simulink model "Nov_27"  (R2022a)
settings: Solver=FixedStepAuto  StartTime=0.0  StopTime=60  FixedStep=1e-3  RelTol=1e-3  EnableMultiTasking=on
undefined symbols (not defined in the file): D0, D1, D10, D11, D12, D13, D2, D3, D4, D5, D6, D7, D8, D9, PTA0, PTA1, PTA2, PTB23, PTB9, PTC16, PTC17, PTC2, PTC3, PTC4, PTD0, PTD1, PTD2, PTD3
libraries: frdmk64flib x16, etargetslib x1
(part 2 of 3)

== stateflow chart Nov_27/Requirements Table ==
  (default) -> (junction 1073743821)
  (junction 1073743821) -> (junction 1073743822) : {
      | % SF_REQ_REV_07
      | }
  (junction 1073743822) -> (junction 1073743824) : {
      | % HEADER_ASSIGNMENTS
      |
      | }
  (junction 1073743824) -> (junction 1073743826) : {
      | % START_A_4
      | }
  (junction 1073743826) -> (junction 1073743828) : {
      | }
  (junction 1073743828) -> (junction 1073743830)
  (junction 1073743830) -> (junction 1073743832) : {
      | }
  (junction 1073743832) -> (junction 1073743834) : {
      | % END_A_4
      | }
  (junction 1073743834) -> (junction 1073743836) : {
      | % START_R_1
      | }
  (junction 1073743836) -> (junction 1073743838) : {
      | }
  (junction 1073743838) -> (junction 1073743840)
  (junction 1073743840) -> (junction 1073743842) [order 1] : [((~((prev(ATR_GND_CTRL)) == (-100.0)))) && ((~((prev(ATR_PACE_CTRL)) == (-100.0)))) && ((~((prev(VENT_PACE_CTRL)) == (-100.0)))) && ((~((prev(VENT_GND_CTRL)) == (-100.0)))) && ((~((prev(PACE_CHARGE_CTRL)) == (-100.0)))) && ((~((VENT_CMP_DETECT) == (true)))) && ((~((ATR_CMP_DETECT) == (true)))) && ((~((VRP) == (-100)))) && (((ARP) == (150)) || ((ARP) == (160)) || ((ARP) == (170)) || ((ARP) == (180)) || ((ARP) == (190)) || ((ARP) == (200)) || ((ARP) == (210)) || ((ARP) == (220)) || ((ARP) == (230)) || ((ARP) == (240)) || ((ARP) == (250)) || ((ARP) == (260)) || ((ARP) == (270)) || ((ARP) == (280)) || ((ARP) == (290)) || ((ARP) == (300)) || ((ARP) == (310)) || ((ARP) == (320)) || ((ARP) == (330)) || ((ARP) == (340)) || ((ARP) == (350)) || ((ARP) == (360)) || ((ARP) == (370)) || ((ARP) == (380)) || ((ARP) == (390)) || ((ARP) == (400)) || ((ARP) == (410)) || ((ARP) == (420)) || ((ARP) == (430)) || ((ARP) == (440)) || ((ARP) == (450)) || ((ARP) == (460)) || ((ARP) == (470)) || ((ARP) == (480)) || ((ARP) == (490)) || ((ARP) == (500))) && (((URL_RATE_LIMIT) == (50)) || ((URL_RATE_LIMIT) == (55)) || ((URL_RATE_LIMIT) == (60)) || ((URL_RATE_LIMIT) == (65)) || ((URL_RATE_LIMIT) == (70)) || ((URL_RATE_LIMIT) == (75)) || ((URL_RATE_LIMIT) == (80)) || ((URL_RATE_LIMIT) == (85)) || ((URL_RATE_LIMIT) == (90)) || ((URL_RATE_LIMIT) == (95)) || ((URL_RATE_LIMIT) == (100)) || ((URL_RATE_LIMIT) == (105)) || ((URL_RATE_LIMIT) == (110)) || ((URL_RATE_LIMIT) == (115)) || ((URL_RATE_LIMIT) == (120)) || ((URL_RATE_LIMIT) == (125)) || ((URL_RATE_LIMIT) == (130)) || ((URL_RATE_LIMIT) == (135)) || ((URL_RATE_LIMIT) == (140)) || ((URL_RATE_LIMIT) == (145)) || ((URL_RATE_LIMIT) == (150)) || ((URL_RATE_LIMIT) == (155)) || ((URL_RATE_LIMIT) == (160)) || ((URL_RATE_LIMIT) == (165)) || ((URL_RATE_LIMIT) == (170)) || ((URL_RATE_LIMIT) == (175))) && (((ATR_PULSE_WIDTH) == (0.05)) || ((ATR_PULSE_WIDTH) == (0.1)) || ((ATR_PULSE_WIDTH) == (0.2)) || ((ATR_PULSE_WIDTH) == (0.3)) || ((ATR_PULSE_WIDTH) == (0.4)) || ((ATR_PULSE_WIDTH) == (0.5)) || ((ATR_PULSE_WIDTH) == (0.6)) || ((ATR_PULSE_WIDTH) == (0.7)) || ((ATR_PULSE_WIDTH) == (0.8)) || ((ATR_PULSE_WIDTH) == (0.9)) || ((ATR_PULSE_WIDTH) == (1)) || ((ATR_PULSE_WIDTH) == (1.1)) || ((ATR_PULSE_WIDTH) == (1.2)) || ((ATR_PULSE_WIDTH) == (1.3)) || ((ATR_PULSE_WIDTH) == (1.4)) || ((ATR_PULSE_WIDTH) == (1.5)) || ((ATR_PULSE_WIDTH) == (1.6)) || ((ATR_PULSE_WIDTH) == (1.7)) || ((ATR_PULSE_WIDTH) == (1.8)) || ((ATR_PULSE_WIDTH) == (1.9))) && ((~((VENT_PULSE_WIDTH) == (-100)))) && (((LRL_RATE_LIMIT) == (30)) || ((LRL_RATE_LIMIT) == (35)) || ((LRL_RATE_LIMIT) == (40)) || ((LRL_RATE_LIMIT) == (45)) || ((LRL_RATE_LIMIT) == (50)) || ((LRL_RATE_LIMIT) == (51)) || ((LRL_RATE_LIMIT) == (52)) || ((LRL_RATE_LIMIT) == (53)) || ((LRL_RATE_LIMIT) == (54)) || ((LRL_RATE_LIMIT) == (55)) || ((LRL_RATE_LIMIT) == (56)) || ((LRL_RATE_LIMIT) == (57)) || ((LRL_RATE_LIMIT) == (58)) || ((LRL_RATE_LIMIT) == (59)) || ((LRL_RATE_LIMIT) == (60)) || ((LRL_RATE_LIMIT) == (61)) || ((LRL_RATE_LIMIT) == (62)) || ((LRL_RATE_LIMIT) == (63)) || ((LRL_RATE_LIMIT) == (64)) || ((LRL_RATE_LIMIT) == (65)) || ((LRL_RATE_LIMIT) == (66)) || ((LRL_RATE_LIMIT) == (67)) || ((LRL_RATE_LIMIT) == (68)) || ((LRL_RATE_LIMIT) == (69)) || ((LRL_RATE_LIMIT) == (70)) || ((LRL_RATE_LIMIT) == (71)) || ((LRL_RATE_LIMIT) == (72)) || ((LRL_RATE_LIMIT) == (73)) || ((LRL_RATE_LIMIT) == (74)) || ((LRL_RATE_LIMIT) == (75)) || ((LRL_RATE_LIMIT) == (76)) || ((LRL_RATE_LIMIT) == (77)) || ((LRL_RATE_LIMIT) == (78)) || ((LRL_RATE_LIMIT) == (79)) || ((LRL_RATE_LIMIT) == (80)) || ((LRL_RATE_LIMIT) == (81)) || ((LRL_RATE_LIMIT) == (82)) || ((LRL_RATE_LIMIT) == (83)) || ((LRL_RATE_LIMIT) == (84)) || ((LRL_RATE_LIMIT) == (85)) || ((LRL_RATE_LIMIT) == (86)) || ((LRL_RATE_LIMIT) == (87)) || ((LRL_RATE_LIMIT) == (88)) || ((LRL_RATE_LIMIT) == (89)) || ((LRL_RATE_LIMIT) == (90)) || ((LRL_RATE_LIMIT) == (95)) || ((LRL_RATE_LIMIT) == (100)) || ((LRL_RATE_LIMIT) == (105)) || ((LRL_RATE_LIMIT) == (110)) || ((LRL_RATE_LIMIT) == (115)) || ((LRL_RATE_LIMIT) == (120)) || ((LRL_RATE_LIMIT) == (125)) || ((LRL_RATE_LIMIT) == (130)) || ((LRL_RATE_LIMIT) == (135)) || ((LRL_RATE_LIMIT) == (140)) || ((LRL_RATE_LIMIT) == (145)) || ((LRL_RATE_LIMIT) == (150)) || ((LRL_RATE_LIMIT) == (155)) || ((LRL_RATE_LIMIT) == (160)) || ((LRL_RATE_LIMIT) == (165)) || ((LRL_RATE_LIMIT) == (170)) || ((LRL_RATE_LIMIT) == (175)))]
  (junction 1073743840) -> (junction 1073743908) [order 2]
  (junction 1073743842) -> (junction 1073743844) : {
      | reqtable_postcondition(((~((ATR_GND_CTRL) == (-100.0)))) && ((~((ATR_PACE_CTRL) == (-100.0)))) && ((~((VENT_PACE_CTRL) == (-100.0)))) && ((~((VENT_GND_CTRL) == (-100.0)))) && ((~((PACE_CHARGE_CTRL) == (-100.0)))), 'R:1');
      |
      |
      | }
  (junction 1073743844) -> (junction 1073743846) : {
      | }
  (junction 1073743846) -> (junction 1073743848) : {
      | sf_internal_execute_R_31 = true;
      | }
  (junction 1073743848) -> (junction 1073743850) : {
      | % START_R_19
      | }
  (junction 1073743850) -> (junction 1073743852) : {
      | }
  (junction 1073743852) -> (junction 1073743854)
  (junction 1073743854) -> (junction 1073743856) [order 1] : [(((prev(ATR_GND_CTRL)) == (true))) && (((prev(ATR_PACE_CTRL)) == (false))) && (((prev(VENT_PACE_CTRL)) == (false))) && (((prev(VENT_GND_CTRL)) == (false))) && (((prev(PACE_CHARGE_CTRL)) == (true))) && ((~((VENT_CMP_DETECT) == (true)))) && ((~((ATR_CMP_DETECT) == (true)))) && ((~((VRP) == (-100)))) && (((ARP) == (150)) || ((ARP) == (160)) || ((ARP) == (170)) || ((ARP) == (180)) || ((ARP) == (190)) || ((ARP) == (200)) || ((ARP) == (210)) || ((ARP) == (220)) || ((ARP) == (230)) || ((ARP) == (240)) || ((ARP) == (250)) || ((ARP) == (260)) || ((ARP) == (270)) || ((ARP) == (280)) || ((ARP) == (290)) || ((ARP) == (300)) || ((ARP) == (310)) || ((ARP) == (320)) || ((ARP) == (330)) || ((ARP) == (340)) || ((ARP) == (350)) || ((ARP) == (360)) || ((ARP) == (370)) || ((ARP) == (380)) || ((ARP) == (390)) || ((ARP) == (400)) || ((ARP) == (410)) || ((ARP) == (420)) || ((ARP) == (430)) || ((ARP) == (440)) || ((ARP) == (450)) || ((ARP) == (460)) || ((ARP) == (470)) || ((ARP) == (480)) || ((ARP) == (490)) || ((ARP) == (500))) && (((URL_RATE_LIMIT) == (50)) || ((URL_RATE_LIMIT) == (55)) || ((URL_RATE_LIMIT) == (60)) || ((URL_RATE_LIMIT) == (65)) || ((URL_RATE_LIMIT) == (70)) || ((URL_RATE_LIMIT) == (75)) || ((URL_RATE_LIMIT) == (80)) || ((URL_RATE_LIMIT) == (85)) || ((URL_RATE_LIMIT) == (90)) || ((URL_RATE_LIMIT) == (95)) || ((URL_RATE_LIMIT) == (100)) || ((URL_RATE_LIMIT) == (105)) || ((URL_RATE_LIMIT) == (110)) || ((URL_RATE_LIMIT) == (115)) || ((URL_RATE_LIMIT) == (120)) || ((URL_RATE_LIMIT) == (125)) || ((URL_RATE_LIMIT) == (130)) || ((URL_RATE_LIMIT) == (135)) || ((URL_RATE_LIMIT) == (140)) || ((URL_RATE_LIMIT) == (145)) || ((URL_RATE_LIMIT) == (150)) || ((URL_RATE_LIMIT) == (155)) || ((URL_RATE_LIMIT) == (160)) || ((URL_RATE_LIMIT) == (165)) || ((URL_RATE_LIMIT) == (170)) || ((URL_RATE_LIMIT) == (175))) && (((ATR_PULSE_WIDTH) == (0.05)) || ((ATR_PULSE_WIDTH) == (0.1)) || ((ATR_PULSE_WIDTH) == (0.2)) || ((ATR_PULSE_WIDTH) == (0.3)) || ((ATR_PULSE_WIDTH) == (0.4)) || ((ATR_PULSE_WIDTH) == (0.5)) || ((ATR_PULSE_WIDTH) == (0.6)) || ((ATR_PULSE_WIDTH) == (0.7)) || ((ATR_PULSE_WIDTH) == (0.8)) || ((ATR_PULSE_WIDTH) == (0.9)) || ((ATR_PULSE_WIDTH) == (1)) || ((ATR_PULSE_WIDTH) == (1.1)) || ((ATR_PULSE_WIDTH) == (1.2)) || ((ATR_PULSE_WIDTH) == (1.3)) || ((ATR_PULSE_WIDTH) == (1.4)) || ((ATR_PULSE_WIDTH) == (1.5)) || ((ATR_PULSE_WIDTH) == (1.6)) || ((ATR_PULSE_WIDTH) == (1.7)) || ((ATR_PULSE_WIDTH) == (1.8)) || ((ATR_PULSE_WIDTH) == (1.9))) && ((~((VENT_PULSE_WIDTH) == (-100)))) && (((LRL_RATE_LIMIT) == (30)) || ((LRL_RATE_LIMIT) == (35)) || ((LRL_RATE_LIMIT) == (40)) || ((LRL_RATE_LIMIT) == (45)) || ((LRL_RATE_LIMIT) == (50)) || ((LRL_RATE_LIMIT) == (51)) || ((LRL_RATE_LIMIT) == (52)) || ((LRL_RATE_LIMIT) == (53)) || ((LRL_RATE_LIMIT) == (54)) || ((LRL_RATE_LIMIT) == (55)) || ((LRL_RATE_LIMIT) == (56)) || ((LRL_RATE_LIMIT) == (57)) || ((LRL_RATE_LIMIT) == (58)) || ((LRL_RATE_LIMIT) == (59)) || ((LRL_RATE_LIMIT) == (60)) || ((LRL_RATE_LIMIT) == (61)) || ((LRL_RATE_LIMIT) == (62)) || ((LRL_RATE_LIMIT) == (63)) || ((LRL_RATE_LIMIT) == (64)) || ((LRL_RATE_LIMIT) == (65)) || ((LRL_RATE_LIMIT) == (66)) || ((LRL_RATE_LIMIT) == (67)) || ((LRL_RATE_LIMIT) == (68)) || ((LRL_RATE_LIMIT) == (69)) || ((LRL_RATE_LIMIT) == (70)) || ((LRL_RATE_LIMIT) == (71)) || ((LRL_RATE_LIMIT) == (72)) || ((LRL_RATE_LIMIT) == (73)) || ((LRL_RATE_LIMIT) == (74)) || ((LRL_RATE_LIMIT) == (75)) || ((LRL_RATE_LIMIT) == (76)) || ((LRL_RATE_LIMIT) == (77)) || ((LRL_RATE_LIMIT) == (78)) || ((LRL_RATE_LIMIT) == (79)) || ((LRL_RATE_LIMIT) == (80)) || ((LRL_RATE_LIMIT) == (81)) || ((LRL_RATE_LIMIT) == (82)) || ((LRL_RATE_LIMIT) == (83)) || ((LRL_RATE_LIMIT) == (84)) || ((LRL_RATE_LIMIT) == (85)) || ((LRL_RATE_LIMIT) == (86)) || ((LRL_RATE_LIMIT) == (87)) || ((LRL_RATE_LIMIT) == (88)) || ((LRL_RATE_LIMIT) == (89)) || ((LRL_RATE_LIMIT) == (90)) || ((LRL_RATE_LIMIT) == (95)) || ((LRL_RATE_LIMIT) == (100)) || ((LRL_RATE_LIMIT) == (105)) || ((LRL_RATE_LIMIT) == (110)) || ((LRL_RATE_LIMIT) == (115)) || ((LRL_RATE_LIMIT) == (120)) || ((LRL_RATE_LIMIT) == (125)) || ((LRL_RATE_LIMIT) == (130)) || ((LRL_RATE_LIMIT) == (135)) || ((LRL_RATE_LIMIT) == (140)) || ((LRL_RATE_LIMIT) == (145)) || ((LRL_RATE_LIMIT) == (150)) || ((LRL_RATE_LIMIT) == (155)) || ((LRL_RATE_LIMIT) == (160)) || ((LRL_RATE_LIMIT) == (165)) || ((LRL_RATE_LIMIT) == (170)) || ((LRL_RATE_LIMIT) == (175)))]
  (junction 1073743854) -> (junction 1073743864) [order 2]
  (junction 1073743856) -> (junction 1073743858) : {
      | reqtable_postcondition((((ATR_GND_CTRL) == (false))) && (((ATR_PACE_CTRL) == (true))) && (((VENT_PACE_CTRL) == (false))) && (((VENT_GND_CTRL) == (false))) && (((PACE_CHARGE_CTRL) == (false))), 'R:1.1');
      |
      |
      | }
  (junction 1073743858) -> (junction 1073743860) : {
      | }
  (junction 1073743860) -> (junction 1073743862) : {
      | sf_internal_execute_R_31 = false;
      | }
  (junction 1073743862) -> (junction 1073743864)
  (junction 1073743864) -> (junction 1073743866)
  (junction 1073743866) -> (junction 1073743868) : {
      | % END_R_19
      | }
  (junction 1073743868) -> (junction 1073743870) : {
      | % START_R_22
      | }
  (junction 1073743870) -> (junction 1073743872) : {
      | }
  (junction 1073743872) -> (junction 1073743874)
  (junction 1073743874) -> (junction 1073743876) [order 1] : [(((prev(ATR_GND_CTRL)) == (true || false))) && (((prev(ATR_PACE_CTRL)) == (true || false))) && (((prev(VENT_PACE_CTRL)) == (false))) && (((prev(VENT_GND_CTRL)) == (false))) && (((prev(PACE_CHARGE_CTRL)) == (true || false))) && ((~((VENT_CMP_DETECT) == (true)))) && (((ATR_CMP_DETECT) == (true))) && ((~((VRP) == (-100)))) && (((ARP) == (150)) || ((ARP) == (160)) || ((ARP) == (170)) || ((ARP) == (180)) || ((ARP) == (190)) || ((ARP) == (200)) || ((ARP) == (210)) || ((ARP) == (220)) || ((ARP) == (230)) || ((ARP) == (240)) || ((ARP) == (250)) || ((ARP) == (260)) || ((ARP) == (270)) || ((ARP) == (280)) || ((ARP) == (290)) || ((ARP) == (300)) || ((ARP) == (310)) || ((ARP) == (320)) || ((ARP) == (330)) || ((ARP) == (340)) || ((ARP) == (350)) || ((ARP) == (360)) || ((ARP) == (370)) || ((ARP) == (380)) || ((ARP) == (390)) || ((ARP) == (400)) || ((ARP) == (410)) || ((ARP) == (420)) || ((ARP) == (430)) || ((ARP) == (440)) || ((ARP) == (450)) || ((ARP) == (460)) || ((ARP) == (470)) || ((ARP) == (480)) || ((ARP) == (490)) || ((ARP) == (500))) && (((URL_RATE_LIMIT) == (50)) || ((URL_RATE_LIMIT) == (55)) || ((URL_RATE_LIMIT) == (60)) || ((URL_RATE_LIMIT) == (65)) || ((URL_RATE_LIMIT) == (70)) || ((URL_RATE_LIMIT) == (75)) || ((URL_RATE_LIMIT) == (80)) || ((URL_RATE_LIMIT) == (85)) || ((URL_RATE_LIMIT) == (90)) || ((URL_RATE_LIMIT) == (95)) || ((URL_RATE_LIMIT) == (100)) || ((URL_RATE_LIMIT) == (105)) || ((URL_RATE_LIMIT) == (110)) || ((URL_RATE_LIMIT) == (115)) || ((URL_RATE_LIMIT) == (120)) || ((URL_RATE_LIMIT) == (125)) || ((URL_RATE_LIMIT) == (130)) || ((URL_RATE_LIMIT) == (135)) || ((URL_RATE_LIMIT) == (140)) || ((URL_RATE_LIMIT) == (145)) || ((URL_RATE_LIMIT) == (150)) || ((URL_RATE_LIMIT) == (155)) || ((URL_RATE_LIMIT) == (160)) || ((URL_RATE_LIMIT) == (165)) || ((URL_RATE_LIMIT) == (170)) || ((URL_RATE_LIMIT) == (175))) && (((ATR_PULSE_WIDTH) == (0.05)) || ((ATR_PULSE_WIDTH) == (0.1)) || ((ATR_PULSE_WIDTH) == (0.2)) || ((ATR_PULSE_WIDTH) == (0.3)) || ((ATR_PULSE_WIDTH) == (0.4)) || ((ATR_PULSE_WIDTH) == (0.5)) || ((ATR_PULSE_WIDTH) == (0.6)) || ((ATR_PULSE_WIDTH) == (0.7)) || ((ATR_PULSE_WIDTH) == (0.8)) || ((ATR_PULSE_WIDTH) == (0.9)) || ((ATR_PULSE_WIDTH) == (1)) || ((ATR_PULSE_WIDTH) == (1.1)) || ((ATR_PULSE_WIDTH) == (1.2)) || ((ATR_PULSE_WIDTH) == (1.3)) || ((ATR_PULSE_WIDTH) == (1.4)) || ((ATR_PULSE_WIDTH) == (1.5)) || ((ATR_PULSE_WIDTH) == (1.6)) || ((ATR_PULSE_WIDTH) == (1.7)) || ((ATR_PULSE_WIDTH) == (1.8)) || ((ATR_PULSE_WIDTH) == (1.9))) && ((~((VENT_PULSE_WIDTH) == (-100)))) && (((LRL_RATE_LIMIT) == (30)) || ((LRL_RATE_LIMIT) == (35)) || ((LRL_RATE_LIMIT) == (40)) || ((LRL_RATE_LIMIT) == (45)) || ((LRL_RATE_LIMIT) == (50)) || ((LRL_RATE_LIMIT) == (51)) || ((LRL_RATE_LIMIT) == (52)) || ((LRL_RATE_LIMIT) == (53)) || ((LRL_RATE_LIMIT) == (54)) || ((LRL_RATE_LIMIT) == (55)) || ((LRL_RATE_LIMIT) == (56)) || ((LRL_RATE_LIMIT) == (57)) || ((LRL_RATE_LIMIT) == (58)) || ((LRL_RATE_LIMIT) == (59)) || ((LRL_RATE_LIMIT) == (60)) || ((LRL_RATE_LIMIT) == (61)) || ((LRL_RATE_LIMIT) == (62)) || ((LRL_RATE_LIMIT) == (63)) || ((LRL_RATE_LIMIT) == (64)) || ((LRL_RATE_LIMIT) == (65)) || ((LRL_RATE_LIMIT) == (66)) || ((LRL_RATE_LIMIT) == (67)) || ((LRL_RATE_LIMIT) == (68)) || ((LRL_RATE_LIMIT) == (69)) || ((LRL_RATE_LIMIT) == (70)) || ((LRL_RATE_LIMIT) == (71)) || ((LRL_RATE_LIMIT) == (72)) || ((LRL_RATE_LIMIT) == (73)) || ((LRL_RATE_LIMIT) == (74)) || ((LRL_RATE_LIMIT) == (75)) || ((LRL_RATE_LIMIT) == (76)) || ((LRL_RATE_LIMIT) == (77)) || ((LRL_RATE_LIMIT) == (78)) || ((LRL_RATE_LIMIT) == (79)) || ((LRL_RATE_LIMIT) == (80)) || ((LRL_RATE_LIMIT) == (81)) || ((LRL_RATE_LIMIT) == (82)) || ((LRL_RATE_LIMIT) == (83)) || ((LRL_RATE_LIMIT) == (84)) || ((LRL_RATE_LIMIT) == (85)) || ((LRL_RATE_LIMIT) == (86)) || ((LRL_RATE_LIMIT) == (87)) || ((LRL_RATE_LIMIT) == (88)) || ((LRL_RATE_LIMIT) == (89)) || ((LRL_RATE_LIMIT) == (90)) || ((LRL_RATE_LIMIT) == (95)) || ((LRL_RATE_LIMIT) == (100)) || ((LRL_RATE_LIMIT) == (105)) || ((LRL_RATE_LIMIT) == (110)) || ((LRL_RATE_LIMIT) == (115)) || ((LRL_RATE_LIMIT) == (120)) || ((LRL_RATE_LIMIT) == (125)) || ((LRL_RATE_LIMIT) == (130)) || ((LRL_RATE_LIMIT) == (135)) || ((LRL_RATE_LIMIT) == (140)) || ((LRL_RATE_LIMIT) == (145)) || ((LRL_RATE_LIMIT) == (150)) || ((LRL_RATE_LIMIT) == (155)) || ((LRL_RATE_LIMIT) == (160)) || ((LRL_RATE_LIMIT) == (165)) || ((LRL_RATE_LIMIT) == (170)) || ((LRL_RATE_LIMIT) == (175)))]
  (junction 1073743874) -> (junction 1073743884) [order 2]
  (junction 1073743876) -> (junction 1073743878) : {
      | reqtable_postcondition((((ATR_GND_CTRL) == (true))) && (((ATR_PACE_CTRL) == (false))) && (((VENT_PACE_CTRL) == (false))) && (((VENT_GND_CTRL) == (false))) && (((PACE_CHARGE_CTRL) == (true))), 'R:1.2');
      |
      |
      | }
  (junction 1073743878) -> (junction 1073743880) : {
      | }
  (junction 1073743880) -> (junction 1073743882) : {
      | sf_internal_execute_R_31 = false;
      | }
  (junction 1073743882) -> (junction 1073743884)
  (junction 1073743884) -> (junction 1073743886)
  (junction 1073743886) -> (junction 1073743888) : {
      | % END_R_22
      | }
  (junction 1073743888) -> (junction 1073743890) : {
      | % START_R_31
      | }
  (junction 1073743890) -> (junction 1073743892) : {
      | }
  (junction 1073743892) -> (junction 1073743894)
  (junction 1073743894) -> (junction 1073743896) [order 1] : [sf_internal_execute_R_31]
  (junction 1073743894) -> (junction 1073743902) [order 2]
  (junction 1073743896) -> (junction 1073743898) : {
      | reqtable_postcondition((((ATR_GND_CTRL) == (true))) && (((ATR_PACE_CTRL) == (false))) && (((VENT_PACE_CTRL) == (false))) && (((VENT_GND_CTRL) == (false))) && (((PACE_CHARGE_CTRL) == (true))), 'R:1.3');
      |
      |
      | }
  (junction 1073743898) -> (junction 1073743900) : {
      | }
  (junction 1073743900) -> (junction 1073743902)
  (junction 1073743902) -> (junction 1073743904)
  (junction 1073743904) -> (junction 1073743906) : {
      | % END_R_31
      | }
  (junction 1073743906) -> (junction 1073743908)
  (junction 1073743908) -> (junction 1073743910)
  (junction 1073743910) -> (junction 1073743912) : {
      | % END_R_1
      | }
  (junction 1073743912) -> (junction 1073743914) : {
      | % START_R_34
      | }
  (junction 1073743914) -> (junction 1073743916) : {
      | }
  (junction 1073743916) -> (junction 1073743918)
  (junction 1073743918) -> (junction 1073743920) [order 1] : [((~((prev(ATR_GND_CTRL)) == (-100.0)))) && ((~((prev(ATR_PACE_CTRL)) == (-100.0)))) && ((~((prev(VENT_PACE_CTRL)) == (-100.0)))) && ((~((prev(VENT_GND_CTRL)) == (-100.0)))) && ((~((prev(PACE_CHARGE_CTRL)) == (-100.0)))) && ((~((VENT_CMP_DETECT) == (true)))) && ((~((ATR_CMP_DETECT) == (true)))) && (((VRP) == (150)) || ((VRP) == (160)) || ((VRP) == (170)) || ((VRP) == (180)) || ((VRP) == (190)) || ((VRP) == (200)) || ((VRP) == (210)) || ((VRP) == (220)) || ((VRP) == (230)) || ((VRP) == (240)) || ((VRP) == (250)) || ((VRP) == (260)) || ((VRP) == (270)) || ((VRP) == (280)) || ((VRP) == (290)) || ((VRP) == (300)) || ((VRP) == (310)) || ((VRP) == (320)) || ((VRP) == (330)) || ((VRP) == (340)) || ((VRP) == (350)) || ((VRP) == (360)) || ((VRP) == (370)) || ((VRP) == (380)) || ((VRP) == (390)) || ((VRP) == (400)) || ((VRP) == (410)) || ((VRP) == (420)) || ((VRP) == (430)) || ((VRP) == (440)) || ((VRP) == (450)) || ((VRP) == (460)) || ((VRP) == (470)) || ((VRP) == (480)) || ((VRP) == (490)) || ((VRP) == (500))) && ((~((ARP) == (-100)))) && (((URL_RATE_LIMIT) == (50)) || ((URL_RATE_LIMIT) == (55)) || ((URL_RATE_LIMIT) == (60)) || ((URL_RATE_LIMIT) == (65)) || ((URL_RATE_LIMIT) == (70)) || ((URL_RATE_LIMIT) == (75)) || ((URL_RATE_LIMIT) == (80)) || ((URL_RATE_LIMIT) == (85)) || ((URL_RATE_LIMIT) == (90)) || ((URL_RATE_LIMIT) == (95)) || ((URL_RATE_LIMIT) == (100)) || ((URL_RATE_LIMIT) == (105)) || ((URL_RATE_LIMIT) == (110)) || ((URL_RATE_LIMIT) == (115)) || ((URL_RATE_LIMIT) == (120)) || ((URL_RATE_LIMIT) == (125)) || ((URL_RATE_LIMIT) == (130)) || ((URL_RATE_LIMIT) == (135)) || ((URL_RATE_LIMIT) == (140)) || ((URL_RATE_LIMIT) == (145)) || ((URL_RATE_LIMIT) == (150)) || ((URL_RATE_LIMIT) == (155)) || ((URL_RATE_LIMIT) == (160)) || ((URL_RATE_LIMIT) == (165)) || ((URL_RATE_LIMIT) == (170)) || ((URL_RATE_LIMIT) == (175))) && ((~((ATR_PULSE_WIDTH) == (-100)))) && (((VENT_PULSE_WIDTH) == (0.05)) || ((VENT_PULSE_WIDTH) == (0.1)) || ((VENT_PULSE_WIDTH) == (0.2)) || ((VENT_PULSE_WIDTH) == (0.3)) || ((VENT_PULSE_WIDTH) == (0.4)) || ((VENT_PULSE_WIDTH) == (0.5)) || ((VENT_PULSE_WIDTH) == (0.6)) || ((VENT_PULSE_WIDTH) == (0.7)) || ((VENT_PULSE_WIDTH) == (0.8)) || ((VENT_PULSE_WIDTH) == (0.9)) || ((VENT_PULSE_WIDTH) == (1)) || ((VENT_PULSE_WIDTH) == (1.1)) || ((VENT_PULSE_WIDTH) == (1.2)) || ((VENT_PULSE_WIDTH) == (1.3)) || ((VENT_PULSE_WIDTH) == (1.4)) || ((VENT_PULSE_WIDTH) == (1.5)) || ((VENT_PULSE_WIDTH) == (1.6)) || ((VENT_PULSE_WIDTH) == (1.7)) || ((VENT_PULSE_WIDTH) == (1.8)) || ((VENT_PULSE_WIDTH) == (1.9))) && (((LRL_RATE_LIMIT) == (30)) || ((LRL_RATE_LIMIT) == (35)) || ((LRL_RATE_LIMIT) == (40)) || ((LRL_RATE_LIMIT) == (45)) || ((LRL_RATE_LIMIT) == (50)) || ((LRL_RATE_LIMIT) == (51)) || ((LRL_RATE_LIMIT) == (52)) || ((LRL_RATE_LIMIT) == (53)) || ((LRL_RATE_LIMIT) == (54)) || ((LRL_RATE_LIMIT) == (55)) || ((LRL_RATE_LIMIT) == (56)) || ((LRL_RATE_LIMIT) == (57)) || ((LRL_RATE_LIMIT) == (58)) || ((LRL_RATE_LIMIT) == (59)) || ((LRL_RATE_LIMIT) == (60)) || ((LRL_RATE_LIMIT) == (61)) || ((LRL_RATE_LIMIT) == (62)) || ((LRL_RATE_LIMIT) == (63)) || ((LRL_RATE_LIMIT) == (64)) || ((LRL_RATE_LIMIT) == (65)) || ((LRL_RATE_LIMIT) == (66)) || ((LRL_RATE_LIMIT) == (67)) || ((LRL_RATE_LIMIT) == (68)) || ((LRL_RATE_LIMIT) == (69)) || ((LRL_RATE_LIMIT) == (70)) || ((LRL_RATE_LIMIT) == (71)) || ((LRL_RATE_LIMIT) == (72)) || ((LRL_RATE_LIMIT) == (73)) || ((LRL_RATE_LIMIT) == (74)) || ((LRL_RATE_LIMIT) == (75)) || ((LRL_RATE_LIMIT) == (76)) || ((LRL_RATE_LIMIT) == (77)) || ((LRL_RATE_LIMIT) == (78)) || ((LRL_RATE_LIMIT) == (79)) || ((LRL_RATE_LIMIT) == (80)) || ((LRL_RATE_LIMIT) == (81)) || ((LRL_RATE_LIMIT) == (82)) || ((LRL_RATE_LIMIT) == (83)) || ((LRL_RATE_LIMIT) == (84)) || ((LRL_RATE_LIMIT) == (85)) || ((LRL_RATE_LIMIT) == (86)) || ((LRL_RATE_LIMIT) == (87)) || ((LRL_RATE_LIMIT) == (88)) || ((LRL_RATE_LIMIT) == (89)) || ((LRL_RATE_LIMIT) == (90)) || ((LRL_RATE_LIMIT) == (95)) || ((LRL_RATE_LIMIT) == (100)) || ((LRL_RATE_LIMIT) == (105)) || ((LRL_RATE_LIMIT) == (110)) || ((LRL_RATE_LIMIT) == (115)) || ((LRL_RATE_LIMIT) == (120)) || ((LRL_RATE_LIMIT) == (125)) || ((LRL_RATE_LIMIT) == (130)) || ((LRL_RATE_LIMIT) == (135)) || ((LRL_RATE_LIMIT) == (140)) || ((LRL_RATE_LIMIT) == (145)) || ((LRL_RATE_LIMIT) == (150)) || ((LRL_RATE_LIMIT) == (155)) || ((LRL_RATE_LIMIT) == (160)) || ((LRL_RATE_LIMIT) == (165)) || ((LRL_RATE_LIMIT) == (170)) || ((LRL_RATE_LIMIT) == (175)))]
  (junction 1073743918) -> (junction 1073743986) [order 2]
  (junction 1073743920) -> (junction 1073743922) : {
      | reqtable_postcondition(((~((ATR_GND_CTRL) == (-100.0)))) && ((~((ATR_PACE_CTRL) == (-100.0)))) && ((~((VENT_PACE_CTRL) == (-100.0)))) && ((~((VENT_GND_CTRL) == (-100.0)))) && ((~((PACE_CHARGE_CTRL) == (-100.0)))), 'R:2');
      |
      |
      | }
  (junction 1073743922) -> (junction 1073743924) : {
      | }
  (junction 1073743924) -> (junction 1073743926) : {
      | sf_internal_execute_R_46 = true;
      | }
  (junction 1073743926) -> (junction 1073743928) : {
      | % START_R_37
      | }
  (junction 1073743928) -> (junction 1073743930) : {
      | }
  (junction 1073743930) -> (junction 1073743932)
  (junction 1073743932) -> (junction 1073743934) [order 1] : [(((prev(ATR_GND_CTRL)) == (false))) && (((prev(ATR_PACE_CTRL)) == (false))) && (((prev(VENT_PACE_CTRL)) == (false))) && (((prev(VENT_GND_CTRL)) == (true))) && (((prev(PACE_CHARGE_CTRL)) == (true))) && ((~((VENT_CMP_DETECT) == (true)))) && ((~((ATR_CMP_DETECT) == (true)))) && (((VRP) == (150)) || ((VRP) == (160)) || ((VRP) == (170)) || ((VRP) == (180)) || ((VRP) == (190)) || ((VRP) == (200)) || ((VRP) == (210)) || ((VRP) == (220)) || ((VRP) == (230)) || ((VRP) == (240)) || ((VRP) == (250)) || ((VRP) == (260)) || ((VRP) == (270)) || ((VRP) == (280)) || ((VRP) == (290)) || ((VRP) == (300)) || ((VRP) == (310)) || ((VRP) == (320)) || ((VRP) == (330)) || ((VRP) == (340)) || ((VRP) == (350)) || ((VRP) == (360)) || ((VRP) == (370)) || ((VRP) == (380)) || ((VRP) == (390)) || ((VRP) == (400)) || ((VRP) == (410)) || ((VRP) == (420)) || ((VRP) == (430)) || ((VRP) == (440)) || ((VRP) == (450)) || ((VRP) == (460)) || ((VRP) == (470)) || ((VRP) == (480)) || ((VRP) == (490)) || ((VRP) == (500))) && ((~((ARP) == (-100)))) && (((URL_RATE_LIMIT) == (50)) || ((URL_RATE_LIMIT) == (55)) || ((URL_RATE_LIMIT) == (60)) || ((URL_RATE_LIMIT) == (65)) || ((URL_RATE_LIMIT) == (70)) || ((URL_RATE_LIMIT) == (75)) || ((URL_RATE_LIMIT) == (80)) || ((URL_RATE_LIMIT) == (85)) || ((URL_RATE_LIMIT) == (90)) || ((URL_RATE_LIMIT) == (95)) || ((URL_RATE_LIMIT) == (100)) || ((URL_RATE_LIMIT) == (105)) || ((URL_RATE_LIMIT) == (110)) || ((URL_RATE_LIMIT) == (115)) || ((URL_RATE_LIMIT) == (120)) || ((URL_RATE_LIMIT) == (125)) || ((URL_RATE_LIMIT) == (130)) || ((URL_RATE_LIMIT) == (135)) || ((URL_RATE_LIMIT) == (140)) || ((URL_RATE_LIMIT) == (145)) || ((URL_RATE_LIMIT) == (150)) || ((URL_RATE_LIMIT) == (155)) || ((URL_RATE_LIMIT) == (160)) || ((URL_RATE_LIMIT) == (165)) || ((URL_RATE_LIMIT) == (170)) || ((URL_RATE_LIMIT) == (175))) && ((~((ATR_PULSE_WIDTH) == (-100)))) && (((VENT_PULSE_WIDTH) == (0.05)) || ((VENT_PULSE_WIDTH) == (0.1)) || ((VENT_PULSE_WIDTH) == (0.2)) || ((VENT_PULSE_WIDTH) == (0.3)) || ((VENT_PULSE_WIDTH) == (0.4)) || ((VENT_PULSE_WIDTH) == (0.5)) || ((VENT_PULSE_WIDTH) == (0.6)) || ((VENT_PULSE_WIDTH) == (0.7)) || ((VENT_PULSE_WIDTH) == (0.8)) || ((VENT_PULSE_WIDTH) == (0.9)) || ((VENT_PULSE_WIDTH) == (1)) || ((VENT_PULSE_WIDTH) == (1.1)) || ((VENT_PULSE_WIDTH) == (1.2)) || ((VENT_PULSE_WIDTH) == (1.3)) || ((VENT_PULSE_WIDTH) == (1.4)) || ((VENT_PULSE_WIDTH) == (1.5)) || ((VENT_PULSE_WIDTH) == (1.6)) || ((VENT_PULSE_WIDTH) == (1.7)) || ((VENT_PULSE_WIDTH) == (1.8)) || ((VENT_PULSE_WIDTH) == (1.9))) && (((LRL_RATE_LIMIT) == (30)) || ((LRL_RATE_LIMIT) == (35)) || ((LRL_RATE_LIMIT) == (40)) || ((LRL_RATE_LIMIT) == (45)) || ((LRL_RATE_LIMIT) == (50)) || ((LRL_RATE_LIMIT) == (51)) || ((LRL_RATE_LIMIT) == (52)) || ((LRL_RATE_LIMIT) == (53)) || ((LRL_RATE_LIMIT) == (54)) || ((LRL_RATE_LIMIT) == (55)) || ((LRL_RATE_LIMIT) == (56)) || ((LRL_RATE_LIMIT) == (57)) || ((LRL_RATE_LIMIT) == (58)) || ((LRL_RATE_LIMIT) == (59)) || ((LRL_RATE_LIMIT) == (60)) || ((LRL_RATE_LIMIT) == (61)) || ((LRL_RATE_LIMIT) == (62)) || ((LRL_RATE_LIMIT) == (63)) || ((LRL_RATE_LIMIT) == (64)) || ((LRL_RATE_LIMIT) == (65)) || ((LRL_RATE_LIMIT) == (66)) || ((LRL_RATE_LIMIT) == (67)) || ((LRL_RATE_LIMIT) == (68)) || ((LRL_RATE_LIMIT) == (69)) || ((LRL_RATE_LIMIT) == (70)) || ((LRL_RATE_LIMIT) == (71)) || ((LRL_RATE_LIMIT) == (72)) || ((LRL_RATE_LIMIT) == (73)) || ((LRL_RATE_LIMIT) == (74)) || ((LRL_RATE_LIMIT) == (75)) || ((LRL_RATE_LIMIT) == (76)) || ((LRL_RATE_LIMIT) == (77)) || ((LRL_RATE_LIMIT) == (78)) || ((LRL_RATE_LIMIT) == (79)) || ((LRL_RATE_LIMIT) == (80)) || ((LRL_RATE_LIMIT) == (81)) || ((LRL_RATE_LIMIT) == (82)) || ((LRL_RATE_LIMIT) == (83)) || ((LRL_RATE_LIMIT) == (84)) || ((LRL_RATE_LIMIT) == (85)) || ((LRL_RATE_LIMIT) == (86)) || ((LRL_RATE_LIMIT) == (87)) || ((LRL_RATE_LIMIT) == (88)) || ((LRL_RATE_LIMIT) == (89)) || ((LRL_RATE_LIMIT) == (90)) || ((LRL_RATE_LIMIT) == (95)) || ((LRL_RATE_LIMIT) == (100)) || ((LRL_RATE_LIMIT) == (105)) || ((LRL_RATE_LIMIT) == (110)) || ((LRL_RATE_LIMIT) == (115)) || ((LRL_RATE_LIMIT) == (120)) || ((LRL_RATE_LIMIT) == (125)) || ((LRL_RATE_LIMIT) == (130)) || ((LRL_RATE_LIMIT) == (135)) || ((LRL_RATE_LIMIT) == (140)) || ((LRL_RATE_LIMIT) == (145)) || ((LRL_RATE_LIMIT) == (150)) || ((LRL_RATE_LIMIT) == (155)) || ((LRL_RATE_LIMIT) == (160)) || ((LRL_RATE_LIMIT) == (165)) || ((LRL_RATE_LIMIT) == (170)) || ((LRL_RATE_LIMIT) == (175)))]
  (junction 1073743932) -> (junction 1073743942) [order 2]
  (junction 1073743934) -> (junction 1073743936) : {
      | reqtable_postcondition((((ATR_GND_CTRL) == (false))) && (((ATR_PACE_CTRL) == (false))) && (((VENT_PACE_CTRL) == (true))) && (((VENT_GND_CTRL) == (false))) && (((PACE_CHARGE_CTRL) == (false))), 'R:2.1');
      |
      |
      | }
  (junction 1073743936) -> (junction 1073743938) : {
      | }
  (junction 1073743938) -> (junction 1073743940) : {
      | sf_internal_execute_R_46 = false;
      | }
  (junction 1073743940) -> (junction 1073743942)
  (junction 1073743942) -> (junction 1073743944)
  (junction 1073743944) -> (junction 1073743946) : {
      | % END_R_37
      | }
  (junction 1073743946) -> (junction 1073743948) : {
      | % START_R_43
      | }
  (junction 1073743948) -> (junction 1073743950) : {
      | }
  (junction 1073743950) -> (junction 1073743952)
  (junction 1073743952) -> (junction 1073743954) [order 1] : [(((prev(ATR_GND_CTRL)) == (false))) && (((prev(ATR_PACE_CTRL)) == (false))) && (((prev(VENT_PACE_CTRL)) == (true || false))) && (((prev(VENT_GND_CTRL)) == (true || false))) && (((prev(PACE_CHARGE_CTRL)) == (true || false))) && (((VENT_CMP_DETECT) == (true))) && ((~((ATR_CMP_DETECT) == (true)))) && (((VRP) == (150)) || ((VRP) == (160)) || ((VRP) == (170)) || ((VRP) == (180)) || ((VRP) == (190)) || ((VRP) == (200)) || ((VRP) == (210)) || ((VRP) == (220)) || ((VRP) == (230)) || ((VRP) == (240)) || ((VRP) == (250)) || ((VRP) == (260)) || ((VRP) == (270)) || ((VRP) == (280)) || ((VRP) == (290)) || ((VRP) == (300)) || ((VRP) == (310)) || ((VRP) == (320)) || ((VRP) == (330)) || ((VRP) == (340)) || ((VRP) == (350)) || ((VRP) == (360)) || ((VRP) == (370)) || ((VRP) == (380)) || ((VRP) == (390)) || ((VRP) == (400)) || ((VRP) == (410)) || ((VRP) == (420)) || ((VRP) == (430)) || ((VRP) == (440)) || ((VRP) == (450)) || ((VRP) == (460)) || ((VRP) == (470)) || ((VRP) == (480)) || ((VRP) == (490)) || ((VRP) == (500))) && ((~((ARP) == (-100)))) && (((URL_RATE_LIMIT) == (50)) || ((URL_RATE_LIMIT) == (55)) || ((URL_RATE_LIMIT) == (60)) || ((URL_RATE_LIMIT) == (65)) || ((URL_RATE_LIMIT) == (70)) || ((URL_RATE_LIMIT) == (75)) || ((URL_RATE_LIMIT) == (80)) || ((URL_RATE_LIMIT) == (85)) || ((URL_RATE_LIMIT) == (90)) || ((URL_RATE_LIMIT) == (95)) || ((URL_RATE_LIMIT) == (100)) || ((URL_RATE_LIMIT) == (105)) || ((URL_RATE_LIMIT) == (110)) || ((URL_RATE_LIMIT) == (115)) || ((URL_RATE_LIMIT) == (120)) || ((URL_RATE_LIMIT) == (125)) || ((URL_RATE_LIMIT) == (130)) || ((URL_RATE_LIMIT) == (135)) || ((URL_RATE_LIMIT) == (140)) || ((URL_RATE_LIMIT) == (145)) || ((URL_RATE_LIMIT) == (150)) || ((URL_RATE_LIMIT) == (155)) || ((URL_RATE_LIMIT) == (160)) || ((URL_RATE_LIMIT) == (165)) || ((URL_RATE_LIMIT) == (170)) || ((URL_RATE_LIMIT) == (175))) && ((~((ATR_PULSE_WIDTH) == (-100)))) && (((VENT_PULSE_WIDTH) == (0.05)) || ((VENT_PULSE_WIDTH) == (0.1)) || ((VENT_PULSE_WIDTH) == (0.2)) || ((VENT_PULSE_WIDTH) == (0.3)) || ((VENT_PULSE_WIDTH) == (0.4)) || ((VENT_PULSE_WIDTH) == (0.5)) || ((VENT_PULSE_WIDTH) == (0.6)) || ((VENT_PULSE_WIDTH) == (0.7)) || ((VENT_PULSE_WIDTH) == (0.8)) || ((VENT_PULSE_WIDTH) == (0.9)) || ((VENT_PULSE_WIDTH) == (1)) || ((VENT_PULSE_WIDTH) == (1.1)) || ((VENT_PULSE_WIDTH) == (1.2)) || ((VENT_PULSE_WIDTH) == (1.3)) || ((VENT_PULSE_WIDTH) == (1.4)) || ((VENT_PULSE_WIDTH) == (1.5)) || ((VENT_PULSE_WIDTH) == (1.6)) || ((VENT_PULSE_WIDTH) == (1.7)) || ((VENT_PULSE_WIDTH) == (1.8)) || ((VENT_PULSE_WIDTH) == (1.9))) && (((LRL_RATE_LIMIT) == (30)) || ((LRL_RATE_LIMIT) == (35)) || ((LRL_RATE_LIMIT) == (40)) || ((LRL_RATE_LIMIT) == (45)) || ((LRL_RATE_LIMIT) == (50)) || ((LRL_RATE_LIMIT) == (51)) || ((LRL_RATE_LIMIT) == (52)) || ((LRL_RATE_LIMIT) == (53)) || ((LRL_RATE_LIMIT) == (54)) || ((LRL_RATE_LIMIT) == (55)) || ((LRL_RATE_LIMIT) == (56)) || ((LRL_RATE_LIMIT) == (57)) || ((LRL_RATE_LIMIT) == (58)) || ((LRL_RATE_LIMIT) == (59)) || ((LRL_RATE_LIMIT) == (60)) || ((LRL_RATE_LIMIT) == (61)) || ((LRL_RATE_LIMIT) == (62)) || ((LRL_RATE_LIMIT) == (63)) || ((LRL_RATE_LIMIT) == (64)) || ((LRL_RATE_LIMIT) == (65)) || ((LRL_RATE_LIMIT) == (66)) || ((LRL_RATE_LIMIT) == (67)) || ((LRL_RATE_LIMIT) == (68)) || ((LRL_RATE_LIMIT) == (69)) || ((LRL_RATE_LIMIT) == (70)) || ((LRL_RATE_LIMIT) == (71)) || ((LRL_RATE_LIMIT) == (72)) || ((LRL_RATE_LIMIT) == (73)) || ((LRL_RATE_LIMIT) == (74)) || ((LRL_RATE_LIMIT) == (75)) || ((LRL_RATE_LIMIT) == (76)) || ((LRL_RATE_LIMIT) == (77)) || ((LRL_RATE_LIMIT) == (78)) || ((LRL_RATE_LIMIT) == (79)) || ((LRL_RATE_LIMIT) == (80)) || ((LRL_RATE_LIMIT) == (81)) || ((LRL_RATE_LIMIT) == (82)) || ((LRL_RATE_LIMIT) == (83)) || ((LRL_RATE_LIMIT) == (84)) || ((LRL_RATE_LIMIT) == (85)) || ((LRL_RATE_LIMIT) == (86)) || ((LRL_RATE_LIMIT) == (87)) || ((LRL_RATE_LIMIT) == (88)) || ((LRL_RATE_LIMIT) == (89)) || ((LRL_RATE_LIMIT) == (90)) || ((LRL_RATE_LIMIT) == (95)) || ((LRL_RATE_LIMIT) == (100)) || ((LRL_RATE_LIMIT) == (105)) || ((LRL_RATE_LIMIT) == (110)) || ((LRL_RATE_LIMIT) == (115)) || ((LRL_RATE_LIMIT) == (120)) || ((LRL_RATE_LIMIT) == (125)) || ((LRL_RATE_LIMIT) == (130)) || ((LRL_RATE_LIMIT) == (135)) || ((LRL_RATE_LIMIT) == (140)) || ((LRL_RATE_LIMIT) == (145)) || ((LRL_RATE_LIMIT) == (150)) || ((LRL_RATE_LIMIT) == (155)) || ((LRL_RATE_LIMIT) == (160)) || ((LRL_RATE_LIMIT) == (165)) || ((LRL_RATE_LIMIT) == (170)) || ((LRL_RATE_LIMIT) == (175)))]
  (junction 1073743952) -> (junction 1073743962) [order 2]
  (junction 1073743954) -> (junction 1073743956) : {
      | reqtable_postcondition((((ATR_GND_CTRL) == (false))) && (((ATR_PACE_CTRL) == (false))) && (((VENT_PACE_CTRL) == (false))) && (((VENT_GND_CTRL) == (true))) && (((PACE_CHARGE_CTRL) == (true))), 'R:2.2');
      |
      |
      | }
  (junction 1073743956) -> (junction 1073743958) : {
      | }
  (junction 1073743958) -> (junction 1073743960) : {
      | sf_internal_execute_R_46 = false;
      | }
  (junction 1073743960) -> (junction 1073743962)
  (junction 1073743962) -> (junction 1073743964)
  (junction 1073743964) -> (junction 1073743966) : {
      | % END_R_43
      | }
  (junction 1073743966) -> (junction 1073743968) : {
      | % START_R_46
      | }
  (junction 1073743968) -> (junction 1073743970) : {
      | }
  (junction 1073743970) -> (junction 1073743972)
  (junction 1073743972) -> (junction 1073743974) [order 1] : [sf_internal_execute_R_46]
  (junction 1073743972) -> (junction 1073743980) [order 2]
  (junction 1073743974) -> (junction 1073743976) : {
      | reqtable_postcondition((((ATR_GND_CTRL) == (false))) && (((ATR_PACE_CTRL) == (false))) && (((VENT_PACE_CTRL) == (false))) && (((VENT_GND_CTRL) == (true))) && (((PACE_CHARGE_CTRL) == (true))), 'R:2.3');
      |
      |
      | }
  (junction 1073743976) -> (junction 1073743978) : {
      | }
  (junction 1073743978) -> (junction 1073743980)
  (junction 1073743980) -> (junction 1073743982)
  (junction 1073743982) -> (junction 1073743984) : {
      | % END_R_46
      | }
  (junction 1073743984) -> (junction 1073743986)
  (junction 1073743986) -> (junction 1073743988)
  (junction 1073743988) -> (junction 1073743990) : {
      | % END_R_34
      | }
  (junction 1073743990) -> (junction 1073743992) : {
      | % START_R_49
      | }
  (junction 1073743992) -> (junction 1073743994) : {
      | }
  (junction 1073743994) -> (junction 1073743996)
  (junction 1073743996) -> (junction 1073743998) [order 1] : [((~((prev(ATR_GND_CTRL)) == (-100.0)))) && ((~((prev(ATR_PACE_CTRL)) == (-100.0)))) && ((~((prev(VENT_PACE_CTRL)) == (-100.0)))) && ((~((prev(VENT_GND_CTRL)) == (-100.0)))) && ((~((prev(PACE_CHARGE_CTRL)) == (-100.0)))) && ((~((VENT_CMP_DETECT) == (true)))) && ((~((ATR_CMP_DETECT) == (true)))) && ((~((VRP) == (-100)))) && ((~((ARP) == (-100)))) && (((URL_RATE_LIMIT) == (50)) || ((URL_RATE_LIMIT) == (55)) || ((URL_RATE_LIMIT) == (60)) || ((URL_RATE_LIMIT) == (65)) || ((URL_RATE_LIMIT) == (70)) || ((URL_RATE_LIMIT) == (75)) || ((URL_RATE_LIMIT) == (80)) || ((URL_RATE_LIMIT) == (85)) || ((URL_RATE_LIMIT) == (90)) || ((URL_RATE_LIMIT) == (95)) || ((URL_RATE_LIMIT) == (100)) || ((URL_RATE_LIMIT) == (105)) || ((URL_RATE_LIMIT) == (110)) || ((URL_RATE_LIMIT) == (115)) || ((URL_RATE_LIMIT) == (120)) || ((URL_RATE_LIMIT) == (125)) || ((URL_RATE_LIMIT) == (130)) || ((URL_RATE_LIMIT) == (135)) || ((URL_RATE_LIMIT) == (140)) || ((URL_RATE_LIMIT) == (145)) || ((URL_RATE_LIMIT) == (150)) || ((URL_RATE_LIMIT) == (155)) || ((URL_RATE_LIMIT) == (160)) || ((URL_RATE_LIMIT) == (165)) || ((URL_RATE_LIMIT) == (170)) || ((URL_RATE_LIMIT) == (175))) && ((~((ATR_PULSE_WIDTH) == (-100)))) && (((VENT_PULSE_WIDTH) == (0.05)) || ((VENT_PULSE_WIDTH) == (0.1)) || ((VENT_PULSE_WIDTH) == (0.2)) || ((VENT_PULSE_WIDTH) == (0.3)) || ((VENT_PULSE_WIDTH) == (0.4)) || ((VENT_PULSE_WIDTH) == (0.5)) || ((VENT_PULSE_WIDTH) == (0.6)) || ((VENT_PULSE_WIDTH) == (0.7)) || ((VENT_PULSE_WIDTH) == (0.8)) || ((VENT_PULSE_WIDTH) == (0.9)) || ((VENT_PULSE_WIDTH) == (1)) || ((VENT_PULSE_WIDTH) == (1.1)) || ((VENT_PULSE_WIDTH) == (1.2)) || ((VENT_PULSE_WIDTH) == (1.3)) || ((VENT_PULSE_WIDTH) == (1.4)) || ((VENT_PULSE_WIDTH) == (1.5)) || ((VENT_PULSE_WIDTH) == (1.6)) || ((VENT_PULSE_WIDTH) == (1.7)) || ((VENT_PULSE_WIDTH) == (1.8)) || ((VENT_PULSE_WIDTH) == (1.9))) && (((LRL_RATE_LIMIT) == (30)) || ((LRL_RATE_LIMIT) == (35)) || ((LRL_RATE_LIMIT) == (40)) || ((LRL_RATE_LIMIT) == (45)) || ((LRL_RATE_LIMIT) == (50)) || ((LRL_RATE_LIMIT) == (51)) || ((LRL_RATE_LIMIT) == (52)) || ((LRL_RATE_LIMIT) == (53)) || ((LRL_RATE_LIMIT) == (54)) || ((LRL_RATE_LIMIT) == (55)) || ((LRL_RATE_LIMIT) == (56)) || ((LRL_RATE_LIMIT) == (57)) || ((LRL_RATE_LIMIT) == (58)) || ((LRL_RATE_LIMIT) == (59)) || ((LRL_RATE_LIMIT) == (60)) || ((LRL_RATE_LIMIT) == (61)) || ((LRL_RATE_LIMIT) == (62)) || ((LRL_RATE_LIMIT) == (63)) || ((LRL_RATE_LIMIT) == (64)) || ((LRL_RATE_LIMIT) == (65)) || ((LRL_RATE_LIMIT) == (66)) || ((LRL_RATE_LIMIT) == (67)) || ((LRL_RATE_LIMIT) == (68)) || ((LRL_RATE_LIMIT) == (69)) || ((LRL_RATE_LIMIT) == (70)) || ((LRL_RATE_LIMIT) == (71)) || ((LRL_RATE_LIMIT) == (72)) || ((LRL_RATE_LIMIT) == (73)) || ((LRL_RATE_LIMIT) == (74)) || ((LRL_RATE_LIMIT) == (75)) || ((LRL_RATE_LIMIT) == (76)) || ((LRL_RATE_LIMIT) == (77)) || ((LRL_RATE_LIMIT) == (78)) || ((LRL_RATE_LIMIT) == (79)) || ((LRL_RATE_LIMIT) == (80)) || ((LRL_RATE_LIMIT) == (81)) || ((LRL_RATE_LIMIT) == (82)) || ((LRL_RATE_LIMIT) == (83)) || ((LRL_RATE_LIMIT) == (84)) || ((LRL_RATE_LIMIT) == (85)) || ((LRL_RATE_LIMIT) == (86)) || ((LRL_RATE_LIMIT) == (87)) || ((LRL_RATE_LIMIT) == (88)) || ((LRL_RATE_LIMIT) == (89)) || ((LRL_RATE_LIMIT) == (90)) || ((LRL_RATE_LIMIT) == (95)) || ((LRL_RATE_LIMIT) == (100)) || ((LRL_RATE_LIMIT) == (105)) || ((LRL_RATE_LIMIT) == (110)) || ((LRL_RATE_LIMIT) == (115)) || ((LRL_RATE_LIMIT) == (120)) || ((LRL_RATE_LIMIT) == (125)) || ((LRL_RATE_LIMIT) == (130)) || ((LRL_RATE_LIMIT) == (135)) || ((LRL_RATE_LIMIT) == (140)) || ((LRL_RATE_LIMIT) == (145)) || ((LRL_RATE_LIMIT) == (150)) || ((LRL_RATE_LIMIT) == (155)) || ((LRL_RATE_LIMIT) == (160)) || ((LRL_RATE_LIMIT) == (165)) || ((LRL_RATE_LIMIT) == (170)) || ((LRL_RATE_LIMIT) == (175)))]
  (junction 1073743996) -> (junction 1073744044) [order 2]
  (junction 1073743998) -> (junction 1073744000) : {
      | reqtable_postcondition(((~((ATR_GND_CTRL) == (-100.0)))) && ((~((ATR_PACE_CTRL) == (-100.0)))) && ((~((VENT_PACE_CTRL) == (-100.0)))) && ((~((VENT_GND_CTRL) == (-100.0)))) && ((~((PACE_CHARGE_CTRL) == (-100.0)))), 'R:3');
      |
      |
      | }
  (junction 1073744000) -> (junction 1073744002) : {
      | }
  (junction 1073744002) -> (junction 1073744004) : {
      | sf_internal_execute_R_55 = true;
      | }
  (junction 1073744004) -> (junction 1073744006) : {
      | % START_R_52
      | }
  (junction 1073744006) -> (junction 1073744008) : {
      | }
  (junction 1073744008) -> (junction 1073744010)
  (junction 1073744010) -> (junction 1073744012) [order 1] : [(((prev(ATR_GND_CTRL)) == (false))) && (((prev(ATR_PACE_CTRL)) == (false))) && (((prev(VENT_PACE_CTRL)) == (false))) && (((prev(VENT_GND_CTRL)) == (true))) && (((prev(PACE_CHARGE_CTRL)) == (true))) && ((~((VENT_CMP_DETECT) == (true)))) && ((~((ATR_CMP_DETECT) == (true)))) && ((~((VRP) == (-100)))) && ((~((ARP) == (-100)))) && (((URL_RATE_LIMIT) == (50)) || ((URL_RATE_LIMIT) == (55)) || ((URL_RATE_LIMIT) == (60)) || ((URL_RATE_LIMIT) == (65)) || ((URL_RATE_LIMIT) == (70)) || ((URL_RATE_LIMIT) == (75)) || ((URL_RATE_LIMIT) == (80)) || ((URL_RATE_LIMIT) == (85)) || ((URL_RATE_LIMIT) == (90)) || ((URL_RATE_LIMIT) == (95)) || ((URL_RATE_LIMIT) == (100)) || ((URL_RATE_LIMIT) == (105)) || ((URL_RATE_LIMIT) == (110)) || ((URL_RATE_LIMIT) == (115)) || ((URL_RATE_LIMIT) == (120)) || ((URL_RATE_LIMIT) == (125)) || ((URL_RATE_LIMIT) == (130)) || ((URL_RATE_LIMIT) == (135)) || ((URL_RATE_LIMIT) == (140)) || ((URL_RATE_LIMIT) == (145)) || ((URL_RATE_LIMIT) == (150)) || ((URL_RATE_LIMIT) == (155)) || ((URL_RATE_LIMIT) == (160)) || ((URL_RATE_LIMIT) == (165)) || ((URL_RATE_LIMIT) == (170)) || ((URL_RATE_LIMIT) == (175))) && ((~((ATR_PULSE_WIDTH) == (-100)))) && (((VENT_PULSE_WIDTH) == (0.05)) || ((VENT_PULSE_WIDTH) == (0.1)) || ((VENT_PULSE_WIDTH) == (0.2)) || ((VENT_PULSE_WIDTH) == (0.3)) || ((VENT_PULSE_WIDTH) == (0.4)) || ((VENT_PULSE_WIDTH) == (0.5)) || ((VENT_PULSE_WIDTH) == (0.6)) || ((VENT_PULSE_WIDTH) == (0.7)) || ((VENT_PULSE_WIDTH) == (0.8)) || ((VENT_PULSE_WIDTH) == (0.9)) || ((VENT_PULSE_WIDTH) == (1)) || ((VENT_PULSE_WIDTH) == (1.1)) || ((VENT_PULSE_WIDTH) == (1.2)) || ((VENT_PULSE_WIDTH) == (1.3)) || ((VENT_PULSE_WIDTH) == (1.4)) || ((VENT_PULSE_WIDTH) == (1.5)) || ((VENT_PULSE_WIDTH) == (1.6)) || ((VENT_PULSE_WIDTH) == (1.7)) || ((VENT_PULSE_WIDTH) == (1.8)) || ((VENT_PULSE_WIDTH) == (1.9))) && (((LRL_RATE_LIMIT) == (30)) || ((LRL_RATE_LIMIT) == (35)) || ((LRL_RATE_LIMIT) == (40)) || ((LRL_RATE_LIMIT) == (45)) || ((LRL_RATE_LIMIT) == (50)) || ((LRL_RATE_LIMIT) == (51)) || ((LRL_RATE_LIMIT) == (52)) || ((LRL_RATE_LIMIT) == (53)) || ((LRL_RATE_LIMIT) == (54)) || ((LRL_RATE_LIMIT) == (55)) || ((LRL_RATE_LIMIT) == (56)) || ((LRL_RATE_LIMIT) == (57)) || ((LRL_RATE_LIMIT) == (58)) || ((LRL_RATE_LIMIT) == (59)) || ((LRL_RATE_LIMIT) == (60)) || ((LRL_RATE_LIMIT) == (61)) || ((LRL_RATE_LIMIT) == (62)) || ((LRL_RATE_LIMIT) == (63)) || ((LRL_RATE_LIMIT) == (64)) || ((LRL_RATE_LIMIT) == (65)) || ((LRL_RATE_LIMIT) == (66)) || ((LRL_RATE_LIMIT) == (67)) || ((LRL_RATE_LIMIT) == (68)) || ((LRL_RATE_LIMIT) == (69)) || ((LRL_RATE_LIMIT) == (70)) || ((LRL_RATE_LIMIT) == (71)) || ((LRL_RATE_LIMIT) == (72)) || ((LRL_RATE_LIMIT) == (73)) || ((LRL_RATE_LIMIT) == (74)) || ((LRL_RATE_LIMIT) == (75)) || ((LRL_RATE_LIMIT) == (76)) || ((LRL_RATE_LIMIT) == (77)) || ((LRL_RATE_LIMIT) == (78)) || ((LRL_RATE_LIMIT) == (79)) || ((LRL_RATE_LIMIT) == (80)) || ((LRL_RATE_LIMIT) == (81)) || ((LRL_RATE_LIMIT) == (82)) || ((LRL_RATE_LIMIT) == (83)) || ((LRL_RATE_LIMIT) == (84)) || ((LRL_RATE_LIMIT) == (85)) || ((LRL_RATE_LIMIT) == (86)) || ((LRL_RATE_LIMIT) == (87)) || ((LRL_RATE_LIMIT) == (88)) || ((LRL_RATE_LIMIT) == (89)) || ((LRL_RATE_LIMIT) == (90)) || ((LRL_RATE_LIMIT) == (95)) || ((LRL_RATE_LIMIT) == (100)) || ((LRL_RATE_LIMIT) == (105)) || ((LRL_RATE_LIMIT) == (110)) || ((LRL_RATE_LIMIT) == (115)) || ((LRL_RATE_LIMIT) == (120)) || ((LRL_RATE_LIMIT) == (125)) || ((LRL_RATE_LIMIT) == (130)) || ((LRL_RATE_LIMIT) == (135)) || ((LRL_RATE_LIMIT) == (140)) || ((LRL_RATE_LIMIT) == (145)) || ((LRL_RATE_LIMIT) == (150)) || ((LRL_RATE_LIMIT) == (155)) || ((LRL_RATE_LIMIT) == (160)) || ((LRL_RATE_LIMIT) == (165)) || ((LRL_RATE_LIMIT) == (170)) || ((LRL_RATE_LIMIT) == (175)))]
  (junction 1073744010) -> (junction 1073744020) [order 2]
  (junction 1073744012) -> (junction 1073744014) : {
      | reqtable_postcondition((((ATR_GND_CTRL) == (false))) && (((ATR_PACE_CTRL) == (false))) && (((VENT_PACE_CTRL) == (true))) && (((VENT_GND_CTRL) == (false))) && (((PACE_CHARGE_CTRL) == (false))), 'R:3.1');
      |
      |
      | }
  (junction 1073744014) -> (junction 1073744016) : {
      | }
  (junction 1073744016) -> (junction 1073744018) : {
      | sf_internal_execute_R_55 = false;
      | }
  (junction 1073744018) -> (junction 1073744020)
  (junction 1073744020) -> (junction 1073744022)
  (junction 1073744022) -> (junction 1073744024) : {
      | % END_R_52
      | }
  (junction 1073744024) -> (junction 1073744026) : {
      | % START_R_55
      | }
  (junction 1073744026) -> (junction 1073744028) : {
      | }
  (junction 1073744028) -> (junction 1073744030)
  (junction 1073744030) -> (junction 1073744032) [order 1] : [sf_internal_execute_R_55]
  (junction 1073744030) -> (junction 1073744038) [order 2]
  (junction 1073744032) -> (junction 1073744034) : {
      | reqtable_postcondition((((ATR_GND_CTRL) == (false))) && (((ATR_PACE_CTRL) == (false))) && (((VENT_PACE_CTRL) == (false))) && (((VENT_GND_CTRL) == (true))) && (((PACE_CHARGE_CTRL) == (true))), 'R:3.2');
      |
      |
      | }
  (junction 1073744034) -> (junction 1073744036) : {
      | }
  (junction 1073744036) -> (junction 1073744038)
  (junction 1073744038) -> (junction 1073744040)
  (junction 1073744040) -> (junction 1073744042) : {
      | % END_R_55
      | }
  (junction 1073744042) -> (junction 1073744044)
  (junction 1073744044) -> (junction 1073744046)
  (junction 1073744046) -> (junction 1073744048) : {
      | % END_R_49
      | }
  (junction 1073744048) -> (junction 1073744050) : {
      | % START_R_58
      | }
  (junction 1073744050) -> (junction 1073744052) : {
      | }
  (junction 1073744052) -> (junction 1073744054)
  (junction 1073744054) -> (junction 1073744056) [order 1] : [((~((prev(ATR_GND_CTRL)) == (-100.0)))) && ((~((prev(ATR_PACE_CTRL)) == (-100.0)))) && ((~((prev(VENT_PACE_CTRL)) == (-100.0)))) && ((~((prev(VENT_GND_CTRL)) == (-100.0)))) && ((~((prev(PACE_CHARGE_CTRL)) == (-100.0)))) && ((~((VENT_CMP_DETECT) == (true)))) && ((~((ATR_CMP_DETECT) == (true)))) && ((~((VRP) == (-100)))) && ((~((ARP) == (-100)))) && (((URL_RATE_LIMIT) == (50)) || ((URL_RATE_LIMIT) == (55)) || ((URL_RATE_LIMIT) == (60)) || ((URL_RATE_LIMIT) == (65)) || ((URL_RATE_LIMIT) == (70)) || ((URL_RATE_LIMIT) == (75)) || ((URL_RATE_LIMIT) == (80)) || ((URL_RATE_LIMIT) == (85)) || ((URL_RATE_LIMIT) == (90)) || ((URL_RATE_LIMIT) == (95)) || ((URL_RATE_LIMIT) == (100)) || ((URL_RATE_LIMIT) == (105)) || ((URL_RATE_LIMIT) == (110)) || ((URL_RATE_LIMIT) == (115)) || ((URL_RATE_LIMIT) == (120)) || ((URL_RATE_LIMIT) == (125)) || ((URL_RATE_LIMIT) == (130)) || ((URL_RATE_LIMIT) == (135)) || ((URL_RATE_LIMIT) == (140)) || ((URL_RATE_LIMIT) == (145)) || ((URL_RATE_LIMIT) == (150)) || ((URL_RATE_LIMIT) == (155)) || ((URL_RATE_LIMIT) == (160)) || ((URL_RATE_LIMIT) == (165)) || ((URL_RATE_LIMIT) == (170)) || ((URL_RATE_LIMIT) == (175))) && (((ATR_PULSE_WIDTH) == (0.05)) || ((ATR_PULSE_WIDTH) == (0.1)) || ((ATR_PULSE_WIDTH) == (0.2)) || ((ATR_PULSE_WIDTH) == (0.3)) || ((ATR_PULSE_WIDTH) == (0.4)) || ((ATR_PULSE_WIDTH) == (0.5)) || ((ATR_PULSE_WIDTH) == (0.6)) || ((ATR_PULSE_WIDTH) == (0.7)) || ((ATR_PULSE_WIDTH) == (0.8)) || ((ATR_PULSE_WIDTH) == (0.9)) || ((ATR_PULSE_WIDTH) == (1)) || ((ATR_PULSE_WIDTH) == (1.1)) || ((ATR_PULSE_WIDTH) == (1.2)) || ((ATR_PULSE_WIDTH) == (1.3)) || ((ATR_PULSE_WIDTH) == (1.4)) || ((ATR_PULSE_WIDTH) == (1.5)) || ((ATR_PULSE_WIDTH) == (1.6)) || ((ATR_PULSE_WIDTH) == (1.7)) || ((ATR_PULSE_WIDTH) == (1.8)) || ((ATR_PULSE_WIDTH) == (1.9))) && ((~((VENT_PULSE_WIDTH) == (-100)))) && (((LRL_RATE_LIMIT) == (30)) || ((LRL_RATE_LIMIT) == (35)) || ((LRL_RATE_LIMIT) == (40)) || ((LRL_RATE_LIMIT) == (45)) || ((LRL_RATE_LIMIT) == (50)) || ((LRL_RATE_LIMIT) == (51)) || ((LRL_RATE_LIMIT) == (52)) || ((LRL_RATE_LIMIT) == (53)) || ((LRL_RATE_LIMIT) == (54)) || ((LRL_RATE_LIMIT) == (55)) || ((LRL_RATE_LIMIT) == (56)) || ((LRL_RATE_LIMIT) == (57)) || ((LRL_RATE_LIMIT) == (58)) || ((LRL_RATE_LIMIT) == (59)) || ((LRL_RATE_LIMIT) == (60)) || ((LRL_RATE_LIMIT) == (61)) || ((LRL_RATE_LIMIT) == (62)) || ((LRL_RATE_LIMIT) == (63)) || ((LRL_RATE_LIMIT) == (64)) || ((LRL_RATE_LIMIT) == (65)) || ((LRL_RATE_LIMIT) == (66)) || ((LRL_RATE_LIMIT) == (67)) || ((LRL_RATE_LIMIT) == (68)) || ((LRL_RATE_LIMIT) == (69)) || ((LRL_RATE_LIMIT) == (70)) || ((LRL_RATE_LIMIT) == (71)) || ((LRL_RATE_LIMIT) == (72)) || ((LRL_RATE_LIMIT) == (73)) || ((LRL_RATE_LIMIT) == (74)) || ((LRL_RATE_LIMIT) == (75)) || ((LRL_RATE_LIMIT) == (76)) || ((LRL_RATE_LIMIT) == (77)) || ((LRL_RATE_LIMIT) == (78)) || ((LRL_RATE_LIMIT) == (79)) || ((LRL_RATE_LIMIT) == (80)) || ((LRL_RATE_LIMIT) == (81)) || ((LRL_RATE_LIMIT) == (82)) || ((LRL_RATE_LIMIT) == (83)) || ((LRL_RATE_LIMIT) == (84)) || ((LRL_RATE_LIMIT) == (85)) || ((LRL_RATE_LIMIT) == (86)) || ((LRL_RATE_LIMIT) == (87)) || ((LRL_RATE_LIMIT) == (88)) || ((LRL_RATE_LIMIT) == (89)) || ((LRL_RATE_LIMIT) == (90)) || ((LRL_RATE_LIMIT) == (95)) || ((LRL_RATE_LIMIT) == (100)) || ((LRL_RATE_LIMIT) == (105)) || ((LRL_RATE_LIMIT) == (110)) || ((LRL_RATE_LIMIT) == (115)) || ((LRL_RATE_LIMIT) == (120)) || ((LRL_RATE_LIMIT) == (125)) || ((LRL_RATE_LIMIT) == (130)) || ((LRL_RATE_LIMIT) == (135)) || ((LRL_RATE_LIMIT) == (140)) || ((LRL_RATE_LIMIT) == (145)) || ((LRL_RATE_LIMIT) == (150)) || ((LRL_RATE_LIMIT) == (155)) || ((LRL_RATE_LIMIT) == (160)) || ((LRL_RATE_LIMIT) == (165)) || ((LRL_RATE_LIMIT) == (170)) || ((LRL_RATE_LIMIT) == (175)))]
  (junction 1073744054) -> (junction 1073744102) [order 2]
  (junction 1073744056) -> (junction 1073744058) : {
      | reqtable_postcondition(((~((ATR_GND_CTRL) == (-100.0)))) && ((~((ATR_PACE_CTRL) == (-100.0)))) && ((~((VENT_PACE_CTRL) == (-100.0)))) && ((~((VENT_GND_CTRL) == (-100.0)))) && ((~((PACE_CHARGE_CTRL) == (-100.0)))), 'R:4');
      |
      |
      | }
  (junction 1073744058) -> (junction 1073744060) : {
      | }
  (junction 1073744060) -> (junction 1073744062) : {
      | sf_internal_execute_R_67 = true;
      | }
  (junction 1073744062) -> (junction 1073744064) : {
      | % START_R_61
      | }
  (junction 1073744064) -> (junction 1073744066) : {
      | }
  (junction 1073744066) -> (junction 1073744068)
  (junction 1073744068) -> (junction 1073744070) [order 1] : [(((prev(ATR_GND_CTRL)) == (true))) && (((prev(ATR_PACE_CTRL)) == (false))) && (((prev(VENT_PACE_CTRL)) == (false))) && (((prev(VENT_GND_CTRL)) == (false))) && (((prev(PACE_CHARGE_CTRL)) == (true))) && ((~((VENT_CMP_DETECT) == (true)))) && ((~((ATR_CMP_DETECT) == (true)))) && ((~((VRP) == (-100)))) && ((~((ARP) == (-100)))) && (((URL_RATE_LIMIT) == (50)) || ((URL_RATE_LIMIT) == (55)) || ((URL_RATE_LIMIT) == (60)) || ((URL_RATE_LIMIT) == (65)) || ((URL_RATE_LIMIT) == (70)) || ((URL_RATE_LIMIT) == (75)) || ((URL_RATE_LIMIT) == (80)) || ((URL_RATE_LIMIT) == (85)) || ((URL_RATE_LIMIT) == (90)) || ((URL_RATE_LIMIT) == (95)) || ((URL_RATE_LIMIT) == (100)) || ((URL_RATE_LIMIT) == (105)) || ((URL_RATE_LIMIT) == (110)) || ((URL_RATE_LIMIT) == (115)) || ((URL_RATE_LIMIT) == (120)) || ((URL_RATE_LIMIT) == (125)) || ((URL_RATE_LIMIT) == (130)) || ((URL_RATE_LIMIT) == (135)) || ((URL_RATE_LIMIT) == (140)) || ((URL_RATE_LIMIT) == (145)) || ((URL_RATE_LIMIT) == (150)) || ((URL_RATE_LIMIT) == (155)) || ((URL_RATE_LIMIT) == (160)) || ((URL_RATE_LIMIT) == (165)) || ((URL_RATE_LIMIT) == (170)) || ((URL_RATE_LIMIT) == (175))) && (((ATR_PULSE_WIDTH) == (0.05)) || ((ATR_PULSE_WIDTH) == (0.1)) || ((ATR_PULSE_WIDTH) == (0.2)) || ((ATR_PULSE_WIDTH) == (0.3)) || ((ATR_PULSE_WIDTH) == (0.4)) || ((ATR_PULSE_WIDTH) == (0.5)) || ((ATR_PULSE_WIDTH) == (0.6)) || ((ATR_PULSE_WIDTH) == (0.7)) || ((ATR_PULSE_WIDTH) == (0.8)) || ((ATR_PULSE_WIDTH) == (0.9)) || ((ATR_PULSE_WIDTH) == (1)) || ((ATR_PULSE_WIDTH) == (1.1)) || ((ATR_PULSE_WIDTH) == (1.2)) || ((ATR_PULSE_WIDTH) == (1.3)) || ((ATR_PULSE_WIDTH) == (1.4)) || ((ATR_PULSE_WIDTH) == (1.5)) || ((ATR_PULSE_WIDTH) == (1.6)) || ((ATR_PULSE_WIDTH) == (1.7)) || ((ATR_PULSE_WIDTH) == (1.8)) || ((ATR_PULSE_WIDTH) == (1.9))) && ((~((VENT_PULSE_WIDTH) == (-100)))) && (((LRL_RATE_LIMIT) == (30)) || ((LRL_RATE_LIMIT) == (35)) || ((LRL_RATE_LIMIT) == (40)) || ((LRL_RATE_LIMIT) == (45)) || ((LRL_RATE_LIMIT) == (50)) || ((LRL_RATE_LIMIT) == (51)) || ((LRL_RATE_LIMIT) == (52)) || ((LRL_RATE_LIMIT) == (53)) || ((LRL_RATE_LIMIT) == (54)) || ((LRL_RATE_LIMIT) == (55)) || ((LRL_RATE_LIMIT) == (56)) || ((LRL_RATE_LIMIT) == (57)) || ((LRL_RATE_LIMIT) == (58)) || ((LRL_RATE_LIMIT) == (59)) || ((LRL_RATE_LIMIT) == (60)) || ((LRL_RATE_LIMIT) == (61)) || ((LRL_RATE_LIMIT) == (62)) || ((LRL_RATE_LIMIT) == (63)) || ((LRL_RATE_LIMIT) == (64)) || ((LRL_RATE_LIMIT) == (65)) || ((LRL_RATE_LIMIT) == (66)) || ((LRL_RATE_LIMIT) == (67)) || ((LRL_RATE_LIMIT) == (68)) || ((LRL_RATE_LIMIT) == (69)) || ((LRL_RATE_LIMIT) == (70)) || ((LRL_RATE_LIMIT) == (71)) || ((LRL_RATE_LIMIT) == (72)) || ((LRL_RATE_LIMIT) == (73)) || ((LRL_RATE_LIMIT) == (74)) || ((LRL_RATE_LIMIT) == (75)) || ((LRL_RATE_LIMIT) == (76)) || ((LRL_RATE_LIMIT) == (77)) || ((LRL_RATE_LIMIT) == (78)) || ((LRL_RATE_LIMIT) == (79)) || ((LRL_RATE_LIMIT) == (80)) || ((LRL_RATE_LIMIT) == (81)) || ((LRL_RATE_LIMIT) == (82)) || ((LRL_RATE_LIMIT) == (83)) || ((LRL_RATE_LIMIT) == (84)) || ((LRL_RATE_LIMIT) == (85)) || ((LRL_RATE_LIMIT) == (86)) || ((LRL_RATE_LIMIT) == (87)) || ((LRL_RATE_LIMIT) == (88)) || ((LRL_RATE_LIMIT) == (89)) || ((LRL_RATE_LIMIT) == (90)) || ((LRL_RATE_LIMIT) == (95)) || ((LRL_RATE_LIMIT) == (100)) || ((LRL_RATE_LIMIT) == (105)) || ((LRL_RATE_LIMIT) == (110)) || ((LRL_RATE_LIMIT) == (115)) || ((LRL_RATE_LIMIT) == (120)) || ((LRL_RATE_LIMIT) == (125)) || ((LRL_RATE_LIMIT) == (130)) || ((LRL_RATE_LIMIT) == (135)) || ((LRL_RATE_LIMIT) == (140)) || ((LRL_RATE_LIMIT) == (145)) || ((LRL_RATE_LIMIT) == (150)) || ((LRL_RATE_LIMIT) == (155)) || ((LRL_RATE_LIMIT) == (160)) || ((LRL_RATE_LIMIT) == (165)) || ((LRL_RATE_LIMIT) == (170)) || ((LRL_RATE_LIMIT) == (175)))]
  (junction 1073744068) -> (junction 1073744078) [order 2]
  (junction 1073744070) -> (junction 1073744072) : {
      | reqtable_postcondition((((ATR_GND_CTRL) == (false))) && (((ATR_PACE_CTRL) == (true))) && (((VENT_PACE_CTRL) == (false))) && (((VENT_GND_CTRL) == (false))) && (((PACE_CHARGE_CTRL) == (false))), 'R:4.1');
      |
      |
      | }
  (junction 1073744072) -> (junction 1073744074) : {
      | }
  (junction 1073744074) -> (junction 1073744076) : {
      | sf_internal_execute_R_67 = false;
      | }
  (junction 1073744076) -> (junction 1073744078)
  (junction 1073744078) -> (junction 1073744080)
  (junction 1073744080) -> (junction 1073744082) : {
      | % END_R_61
      | }
  (junction 1073744082) -> (junction 1073744084) : {
      | % START_R_67
      | }
  (junction 1073744084) -> (junction 1073744086) : {
      | }
  (junction 1073744086) -> (junction 1073744088)
  (junction 1073744088) -> (junction 1073744090) [order 1] : [sf_internal_execute_R_67]
  (junction 1073744088) -> (junction 1073744096) [order 2]
  (junction 1073744090) -> (junction 1073744092) : {
      | reqtable_postcondition((((ATR_GND_CTRL) == (true))) && (((ATR_PACE_CTRL) == (false))) && (((VENT_PACE_CTRL) == (false))) && (((VENT_GND_CTRL) == (false))) && (((PACE_CHARGE_CTRL) == (true))), 'R:4.2');
      |
      |
      | }
  (junction 1073744092) -> (junction 1073744094) : {
      | }
  (junction 1073744094) -> (junction 1073744096)
  (junction 1073744096) -> (junction 1073744098)
  (junction 1073744098) -> (junction 1073744100) : {
      | % END_R_67
      | }
  (junction 1073744100) -> (junction 1073744102)
  (junction 1073744102) -> (junction 1073744104)
  (junction 1073744104) -> (junction 1073744106) : {
      | % END_R_58
      | }
  data: LRL_RATE_LIMIT input; URL_RATE_LIMIT input; VENT_PULSE_WIDTH input; ATR_PULSE_WIDTH input; VRP input; ARP input; VENT_CMP_DETECT input; ATR_CMP_DETECT input; VENT_GND_CTRL input; VENT_PACE_CTRL input; ATR_GND_CTRL input; PACE_CHARGE_CTRL input; ATR_PACE_CTRL input
